simulink model "toApp"  (R2020a)
settings: Solver=ode3  StartTime=0.0  StopTime=inf  RelTol=1e-3
undefined symbols (not defined in the file): fdesignblkfcn, gcbh
libraries: androidsensorlib x1, dspmlti4 x1, realtime_examples_misc x1, androidadvancedlib x1
PreSaveFcn:
  | set_param(gcs, 'Location',[35 56 895 605])
settings Model: ExtModeTrigDuration=100  Creator=The MathWorks, Inc.  LastModifiedBy=luisi
settings DataIOCC: LimitDataPoints=on  SaveFormat=Array  ReturnWorkspaceOutputs=off
settings OptimizationCC: LifeSpan=Inf  MaxStackSize=64
settings DebuggingCC: UnderspecifiedInitializationDetection=Classic  MergeDetectMultiDrivingBlocksExec=none  ParameterPrecisionLossMsg=none  AllowSymbolicDim=off  SymbolicDimsDataTypeCodeGenerationDiagnostic=none  SFUnexpectedBacktrackingDiag=warning  SFNoUnconditionalDefaultTransitionDiag=warning  SFExecutionAtInitializationDiag=none  ArithmeticOperatorsInVariantConditions=warning
settings HardwareCC: ProdBitPerPointer=32  ProdLargestAtomicInteger=Long  ProdLargestAtomicFloat=Double  ProdWordSize=32  ProdHWDeviceType=ARM Compatible->ARM Cortex  TargetLargestAtomicInteger=Long  TargetLargestAtomicFloat=Double  TargetEndianess=LittleEndian  TargetHWDeviceType=ARM Compatible->ARM Cortex  UseEmbeddedCoderFeatures=off  UseSimulinkCoderFeatures=off
settings ModelReferenceCC: PropagateSignalLabelsOutOfModel=off
settings SFSimCC: SimUseLocalCustomCode=off  CustomCodeUndefinedFunction=UseInterfaceOnly
settings RTWCC: SystemTargetFile=ert.tlc  HardwareBoard=Android Device  TemplateMakefile=ert_default_tmf  GenerateReport=on  RTWVerbose=off  RTWUseLocalCustomCode=off  Toolchain=Android SDK/NDK Tools  LaunchReport=on
settings CodeAppCC: ForceParamTrailComments=on  OperatorAnnotations=on  StateflowObjectComments=on  MATLABSourceComments=on
settings ERTTargetCC: MultiwordLength=2048  ERTCustomFileBanners=off  SupportContinuousTime=on  SupportNonInlinedSFcns=on  RemoveResetFunc=off  ModelStepFunctionPrototypeControlCompliant=off
settings ConfigComp: CovMetricSettings=dw  CovHtmlReporting=on  CovSaveCumulativeToWorkspaceVar=on  CovSaveSingleToWorkspaceVar=on  CovExternalEMLEnable=off  CovSFcnEnable=off

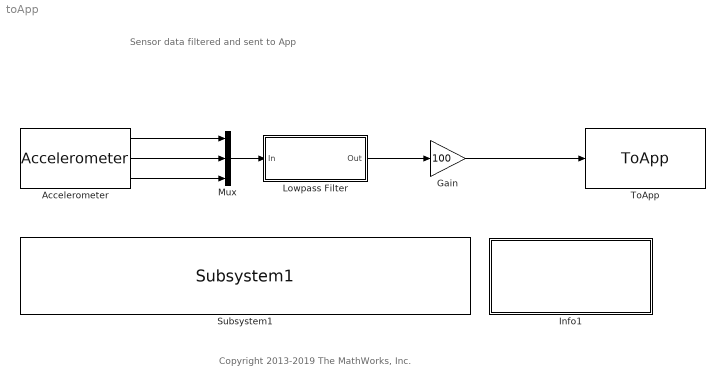
== system toApp ==
  note: Copyright 2013-2019 The MathWorks, Inc.
  note: Sensor data filtered and sent to App
  Accelerometer : androidsensorlib/Accelerometer  OutputVector=off  SampleTime=0.1  BlockPlatform=Android
      settings: SourceProductBaseCode=ANDROID
  Gain : Gain  Gain=100
  Info1 : Subsystem  Description=Descibes demo and operating procedure.
      settings: OpenFcn=android_updatesensorapplication(bdroot);
      mask Display: fprintf('Double click this block to\nupdate the application\nwith animation')
  Lowpass Filter : Subsystem  DialogController=fdesignblkfcn  InitFcn=fdesignblkfcn(gcbh, {'InitFcn'});  mask(Lowpass Filter){}
      mask help: Design a lowpass filter
      settings: CopyFcn=fdesignblkfcn(gcbh, {'CopyFcn'});
      mask Help: helpview(mapfilelocation('dsp'), 'dsplowpassfilter');
      mask Display: disp('Lowpass')
  Mux : Mux  Inputs=3
  Subsystem1 : realtime_examples_misc/Subsystem1  SystemSampleTime=-1  Latency=0  AutoFrameSizeCalculation=off
      settings: SourceProductBaseCode=SL
  ToApp : androidadvancedlib/ToApp  FunctionName=FilteredData  NumInputs=1
      settings: SourceProductBaseCode=ANDROID
  wires:
  Mux/1 -> Lowpass Filter/1(In)
  Accelerometer/1 -> Mux/1
  Accelerometer/3 -> Mux/3
  Accelerometer/2 -> Mux/2
  Lowpass Filter/1(Out) -> Gain/1
  Gain/1 -> ToApp/1

== system toApp/Info1 ==

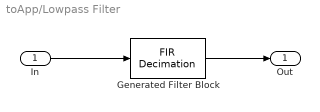
== system toApp/Lowpass Filter ==
  In : Inport
  Generated Filter Block : dspmlti4/FIR Decimation  Tag=BlockMethodSubSystem  FilterSource=Dialog parameters  h=[-0.0010231845453564916 -0.0014087999050194434 -0.0021662168058524693 -0.0029673825521073422 -0.0036809535691406689 -0.0041433880931616117 -0.0041810904868763111 -0.0036398757865999305 -0.0024201621664476708 -0.00050885124287957436 0.0019956674929653469 0.0048722653087206434 0.0077837786847600931 0.010309385048913426 0.011994146569776562 0.012415175398684745 0.011256274500360043 0.0083833045612758342 0.0038964246132389621 -0.0018343193373245061 -0.0081735933482507944 -0.014267318118257988 -0.019118627612890741 -0.021705777573646997 -0.021108471293099385 -0.016644260301461409 -0.0079813005503426328 0.0047775786678150413 0.02106350746186544 0.039864670368991967 0.059808452765460422 0.07929145941585411 0.096648169895404229 0.11033117628061295 0.11908731352350241 0.12210005725715639 0.11908731352350241 0.11033117628061295 0.096648169895404229 0.07929145941585411 0.059808452765460422 0.039864670368991967 0.02106350746186544 0.0047775786678150413 -0.0079813005503426328 -0.016644260301461409 -0.021108471293099385 -0.021705777573646997 -0.019118627612890741 -0.014267318118257988 -0.0081735933482507944 -0.0018343193373245061 0.0038964246132389621 0.0083833045612758342 0.011256274500360043 0.012415175398684745 0.011994146569776562 0.010309385048913426 0.0077837786847600931 0.0048722653087206434 0.0019956674929653469 -0.00050885124287957436 -0.0024201621664476708 -0.0036398757865999305 -0.0041810904868763111 -0.0041433880931616117 -0.0036809535691406689 -0.0029673825521073422 -0.0021662168058524693 -0.0014087999050194434 -0.0010231845453564916]  D=2  filtStruct=Direct form  FilterObject=Hm_firdecim  framing=Allow multirate processing  inputOffset=0  outputBufInitCond=0  roundingMode=Floor  overflowMode=off  firstCoeffDataTypeStr=Inherit: Same word length as input  firstCoeffMin=[]  firstCoeffMax=[]  firstCoeffLastDataTypeStr=Inherit: Same word length as input  outputDataTypeStr=Inherit: Same as accumulator  outputMin=[]  outputMax=[]  outputLastDataTypeStr=Inherit: Same as accumulator
  Out : Outport  VectorParamsAs1DForOutWhenUnconnected=off
  wires:
  Generated Filter Block/1 -> Out/1
  In/1 -> Generated Filter Block/1
